simulink model "w1p3"  (R2020b)
settings: Solver=VariableStepAuto  StartTime=0.0  StopTime=10  MaxStep=0.0001  RelTol=1e-3
settings Model: Creator=Dell  LastModifiedBy=Dell

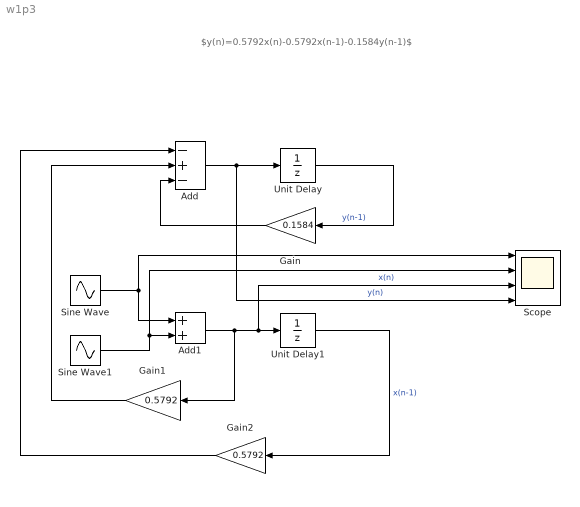
== system w1p3 ==
  note: $y(n)=0.5792x(n)-0.5792x(n-1)-0.1584y(n-1)$
  Add : Sum  Inputs=-+-
  Add1 : Sum
  Gain : Gain  Gain=0.1584
  Gain1 : Gain  Gain=0.5792
  Gain2 : Gain  Gain=0.5792
  Scope : Scope  NumInputPorts=4
  Sine Wave : Sin  Frequency=400  SampleTime=0
  Sine Wave1 : Sin  Frequency=4000  SampleTime=0
  Unit Delay : UnitDelay  SampleTime=-1  HasFrameUpgradeWarning=on
  Unit Delay1 : UnitDelay  SampleTime=-1  HasFrameUpgradeWarning=on
  wires:
  Add/1 -> Scope/4, Unit Delay/1  "y(n)"
  Unit Delay/1 -> Gain/1  "y(n-1)"
  Gain/1 -> Add/3
  Add1/1 -> Scope/3, Unit Delay1/1, Gain1/1  "x(n)"
  Sine Wave/1 -> Scope/1, Add1/1
  Sine Wave1/1 -> Scope/2, Add1/2
  Unit Delay1/1 -> Gain2/1  "x(n-1)"
  Gain1/1 -> Add/2
  Gain2/1 -> Add/1
